simulink model "StimaFrenquenza_2"  (R2019b)
settings: Solver=ode15s  StartTime=0.0  StopTime=50  MaxStep=1e-3  RelTol=1e-3
undefined symbols (not defined in the file or in its folder): h, h2, st, tau_max
libraries: fl_lib x13, nesl_utility x8, simulink x3
settings Model: OrderedModelArguments=off  Creator=manue  LastModifiedBy=manue
settings DataIOCC: SaveFormat=StructureWithTime

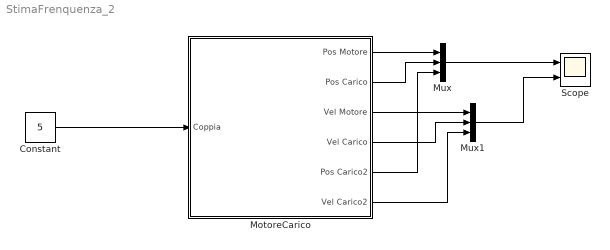
== system StimaFrenquenza_2 ==
  Constant : Constant  Value=5
  MotoreCarico : Subsystem
  Mux : Mux  Inputs=3
  Mux1 : Mux  Inputs=3
  Scope : Scope  NumInputPorts=2
  wires:
  MotoreCarico/1(Pos Motore) -> Mux/1
  MotoreCarico/2(Pos Carico) -> Mux/2
  Mux/1 -> Scope/1
  MotoreCarico/3(Vel Motore) -> Mux1/1
  MotoreCarico/4(Vel Carico) -> Mux1/2
  Mux1/1 -> Scope/2
  Constant/1 -> MotoreCarico/1(Coppia)
  MotoreCarico/5(Pos Carico2) -> Mux/3
  MotoreCarico/6(Vel Carico2) -> Mux1/3

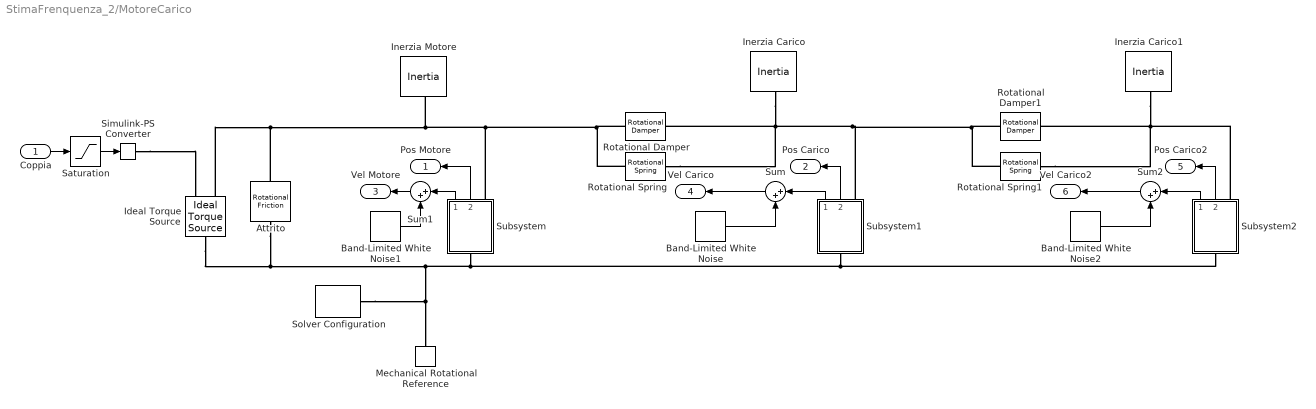
== system StimaFrenquenza_2/MotoreCarico ==
  Coppia : Inport
  Attrito : fl_lib/Mechanical/Rotational Elements/Rotational Friction  brkwy_trq=Fc N*m  brkwy_vel=0.1 rad/s  Col_trq=Fc N*m  visc_coef=Fv N*m/(rad/s)  w_specify=off  w_priority=None  w=0 rad/s  w_nominal_specify=off  w_nominal_unit=rad/s  w_nominal_value=1  t_specify=off  t_priority=None  t=0 N*m  t_nominal_specify=off  t_nominal_unit=N*m  t_nominal_value=1
      settings: SourceProductName=Simscape
  Band-Limited White Noise : simulink/Sources/Band-Limited White Noise  Cov=0.00000001  Ts=st  seed=[23341]
  Band-Limited White Noise1 : simulink/Sources/Band-Limited White Noise  Cov=0.00000001  Ts=st  seed=[23341]
  Band-Limited White Noise2 : simulink/Sources/Band-Limited White Noise  Cov=0.00000001  Ts=st  seed=[23341]
  Ideal Torque Source : fl_lib/Mechanical/Mechanical Sources/Ideal Torque Source
  Inerzia Carico : fl_lib/Mechanical/Rotational Elements/Inertia  inertia=Jc kg*m^2  w_specify=off  w_priority=High  w=0 rad/s  w_nominal_specify=off  w_nominal_unit=rad/s  w_nominal_value=1  t_specify=off  t_priority=None  t=0 N*m  t_nominal_specify=off  t_nominal_unit=N*m  t_nominal_value=1
  Inerzia Carico1 : fl_lib/Mechanical/Rotational Elements/Inertia  inertia=Jc kg*m^2  w_specify=off  w_priority=High  w=0 rad/s  w_nominal_specify=off  w_nominal_unit=rad/s  w_nominal_value=1  t_specify=off  t_priority=None  t=0 N*m  t_nominal_specify=off  t_nominal_unit=N*m  t_nominal_value=1
  Inerzia Motore : fl_lib/Mechanical/Rotational Elements/Inertia  inertia=Jm kg*m^2  w_specify=off  w_priority=High  w=0 rad/s  w_nominal_specify=off  w_nominal_unit=rad/s  w_nominal_value=1  t_specify=off  t_priority=None  t=0 N*m  t_nominal_specify=off  t_nominal_unit=N*m  t_nominal_value=1
  Mechanical Rotational Reference : fl_lib/Mechanical/Rotational Elements/Mechanical Rotational Reference
  Rotational Damper : fl_lib/Mechanical/Rotational Elements/Rotational Damper  D=h N*m/(rad/s)  w_specify=off  w_priority=None  w=0 rad/s  w_nominal_specify=off  w_nominal_unit=rad/s  w_nominal_value=1  t_specify=off  t_priority=None  t=0 N*m  t_nominal_specify=off  t_nominal_unit=N*m  t_nominal_value=1
  Rotational Damper1 : fl_lib/Mechanical/Rotational Elements/Rotational Damper  D=h2 N*m/(rad/s)  w_specify=off  w_priority=None  w=0 rad/s  w_nominal_specify=off  w_nominal_unit=rad/s  w_nominal_value=1  t_specify=off  t_priority=None  t=0 N*m  t_nominal_specify=off  t_nominal_unit=N*m  t_nominal_value=1
  Rotational Spring : fl_lib/Mechanical/Rotational Elements/Rotational Spring  spr_rate=k N*m/rad  w_specify=off  w_priority=None  w=0 rad/s  w_nominal_specify=off  w_nominal_unit=rad/s  w_nominal_value=1  t_specify=off  t_priority=None  t=0 N*m  t_nominal_specify=off  t_nominal_unit=N*m  t_nominal_value=1  phi_specify=off  phi_priority=High  phi=0 rad  phi_nominal_specify=off  phi_nominal_unit=rad  phi_nominal_value=1
      settings: SourceProductName=Simscape
  Rotational Spring1 : fl_lib/Mechanical/Rotational Elements/Rotational Spring  spr_rate=k2 N*m/rad  w_specify=off  w_priority=None  w=0 rad/s  w_nominal_specify=off  w_nominal_unit=rad/s  w_nominal_value=1  t_specify=off  t_priority=None  t=0 N*m  t_nominal_specify=off  t_nominal_unit=N*m  t_nominal_value=1  phi_specify=off  phi_priority=High  phi=0 rad  phi_nominal_specify=off  phi_nominal_unit=rad  phi_nominal_value=1
      settings: SourceProductName=Simscape
  Saturation : Saturate  UpperLimit=tau_max  LowerLimit=-tau_max
  Simulink-PS Converter : nesl_utility/Simulink-PS Converter  PhysicalDomain=network_engine_domain  SubClassName=ps_input  LeftPortType=input  RightPortType=output  PseudoPeriodic=off  Frequencies=[]  NoiseDistribution=none  NoiseParameters=[]  Unit=1  AffineConversion=off  FilteringAndDerivatives=provide  SimscapeFilterOrder=1  InputFilterTimeConstant=0.001  UdotUserProvided=0
  Solver Configuration : nesl_utility/Solver Configuration  PhysicalDomain=network_engine_domain  SubClassName=solver  LeftPortType=input  RightPortType=generic  Tones=[]  Harmonics=[]  SimulateNoise=off  Profile=off  UseLocalSampling=off  EnableSwitchedLinearOptims=on  FrequencyDomain=off  UseCCode=off  RelTol=0.001  AbsTol=1e-06  MinStep=1e-09  ToWorkspace=off  RevertToSquareIcSolve=off  NumHomotopyIterations=100  PhasorMode=off  PhasorModeNumHarmonics=1  DoDC=off  ResidualTolerance=1e-09  UseLocalSolver=off  LocalSolverChoice=NE_BACKWARD_EULER_ADVANCER  LocalSolverSampleTime=0.001  DoFixedCost=off  MaxNonlinIter=3  MaxModeIter=2  LinearAlgebra=auto  EquationFormulation=NE_TIME_EF  DelaysMemoryBudget=1024  AutomaticFiltering=on  FilteringTimeConstant=0.001  PartitionStorageMethod=AS_NEEDED  PartitionMemoryBudget=1024  PartitionMethod=ROBUST
  Subsystem : Subsystem
  Subsystem1 : Subsystem
  Subsystem2 : Subsystem
  Sum : Sum  Inputs=|++
  Sum1 : Sum  Inputs=|++
  Sum2 : Sum  Inputs=|++
  Pos Motore : Outport
  Pos Carico : Outport  Port=2
  Vel Motore : Outport  Port=3
  Vel Carico : Outport  Port=4
  Pos Carico2 : Outport  Port=5
  Vel Carico2 : Outport  Port=6
  wires:
  Coppia/1 -> Saturation/1
  Subsystem/1(Velocity) -> Sum1/1
  Subsystem1/1(Velocity) -> Sum/1
  Subsystem/2(Position) -> Pos Motore/1
  Subsystem1/2(Position) -> Pos Carico/1
  Sum/1 -> Vel Carico/1
  Band-Limited White Noise/1 -> Sum/2
  Sum1/1 -> Vel Motore/1
  Band-Limited White Noise1/1 -> Sum1/2
  Saturation/1 -> Simulink-PS Converter/1
  Subsystem2/2(Position) -> Pos Carico2/1
  Band-Limited White Noise2/1 -> Sum2/2
  Subsystem2/1(Velocity) -> Sum2/1
  Sum2/1 -> Vel Carico2/1
  connections:
  Ideal Torque Source/LConn1 -- Attrito/LConn1 -- Subsystem2/LConn1 -- Subsystem1/LConn1 -- Subsystem/LConn1 -- Solver Configuration/RConn1 -- Mechanical Rotational Reference/LConn1
  Simulink-PS Converter/RConn1 -- Ideal Torque Source/RConn1
  Ideal Torque Source/RConn2 -- Attrito/RConn1 -- Rotational Spring/LConn1 -- Rotational Damper/LConn1 -- Subsystem/RConn1 -- Inerzia Motore/LConn1
  Rotational Damper1/LConn1 -- Inerzia Carico/LConn1 -- Rotational Spring/RConn1 -- Rotational Damper/RConn1 -- Subsystem1/RConn1 -- Rotational Spring1/LConn1
  Rotational Damper1/RConn1 -- Inerzia Carico1/LConn1 -- Rotational Spring1/RConn1 -- Subsystem2/RConn1

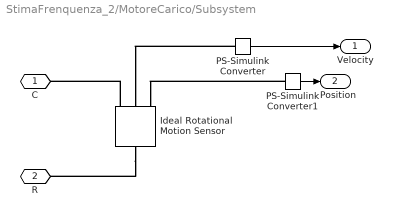
== system StimaFrenquenza_2/MotoreCarico/Subsystem ==
  Ideal Rotational Motion Sensor : fl_lib/Mechanical/Mechanical Sensors/Ideal Rotational Motion Sensor  offset=0 rad
  PS-Simulink Converter : nesl_utility/PS-Simulink Converter  PhysicalDomain=network_engine_domain  SubClassName=ps_output  LeftPortType=input  RightPortType=output  PseudoPeriodic=off  Frequencies=[]  Unit=inherit  AffineConversion=off
  PS-Simulink Converter1 : nesl_utility/PS-Simulink Converter  PhysicalDomain=network_engine_domain  SubClassName=ps_output  LeftPortType=input  RightPortType=output  PseudoPeriodic=off  Frequencies=[]  Unit=inherit  AffineConversion=off
  C : PMIOPort  Side=Right
  R : PMIOPort  Port=2  Side=Left
  Velocity : Outport
  Position : Outport  Port=2
  wires:
  PS-Simulink Converter/1 -> Velocity/1
  PS-Simulink Converter1/1 -> Position/1
  connections:
  PS-Simulink Converter1/LConn1 -- Ideal Rotational Motion Sensor/RConn3
  Ideal Rotational Motion Sensor/LConn1 -- R/RConn1
  PS-Simulink Converter/LConn1 -- Ideal Rotational Motion Sensor/RConn2
  Ideal Rotational Motion Sensor/RConn1 -- C/RConn1

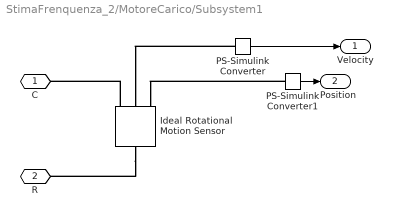
== system StimaFrenquenza_2/MotoreCarico/Subsystem1 ==
  Ideal Rotational Motion Sensor : fl_lib/Mechanical/Mechanical Sensors/Ideal Rotational Motion Sensor  offset=0 rad
  PS-Simulink Converter : nesl_utility/PS-Simulink Converter  PhysicalDomain=network_engine_domain  SubClassName=ps_output  LeftPortType=input  RightPortType=output  PseudoPeriodic=off  Frequencies=[]  Unit=inherit  AffineConversion=off
  PS-Simulink Converter1 : nesl_utility/PS-Simulink Converter  PhysicalDomain=network_engine_domain  SubClassName=ps_output  LeftPortType=input  RightPortType=output  PseudoPeriodic=off  Frequencies=[]  Unit=inherit  AffineConversion=off
  C : PMIOPort  Side=Right
  R : PMIOPort  Port=2  Side=Left
  Velocity : Outport
  Position : Outport  Port=2
  wires:
  PS-Simulink Converter1/1 -> Position/1
  PS-Simulink Converter/1 -> Velocity/1
  connections:
  Ideal Rotational Motion Sensor/RConn1 -- C/RConn1
  PS-Simulink Converter/LConn1 -- Ideal Rotational Motion Sensor/RConn2
  Ideal Rotational Motion Sensor/LConn1 -- R/RConn1
  PS-Simulink Converter1/LConn1 -- Ideal Rotational Motion Sensor/RConn3

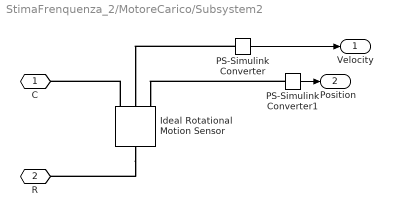
== system StimaFrenquenza_2/MotoreCarico/Subsystem2 ==
  Ideal Rotational Motion Sensor : fl_lib/Mechanical/Mechanical Sensors/Ideal Rotational Motion Sensor  offset=0 rad
  PS-Simulink Converter : nesl_utility/PS-Simulink Converter  PhysicalDomain=network_engine_domain  SubClassName=ps_output  LeftPortType=input  RightPortType=output  PseudoPeriodic=off  Frequencies=[]  Unit=inherit  AffineConversion=off
  PS-Simulink Converter1 : nesl_utility/PS-Simulink Converter  PhysicalDomain=network_engine_domain  SubClassName=ps_output  LeftPortType=input  RightPortType=output  PseudoPeriodic=off  Frequencies=[]  Unit=inherit  AffineConversion=off
  C : PMIOPort  Side=Right
  R : PMIOPort  Port=2  Side=Left
  Velocity : Outport
  Position : Outport  Port=2
  wires:
  PS-Simulink Converter1/1 -> Position/1
  PS-Simulink Converter/1 -> Velocity/1
  connections:
  Ideal Rotational Motion Sensor/RConn1 -- C/RConn1
  PS-Simulink Converter/LConn1 -- Ideal Rotational Motion Sensor/RConn2
  Ideal Rotational Motion Sensor/LConn1 -- R/RConn1
  PS-Simulink Converter1/LConn1 -- Ideal Rotational Motion Sensor/RConn3
